simulink model "Zad_3_sch"  (R2022a)
settings: Solver=VariableStepAuto  StartTime=0.0  StopTime=10.0  RelTol=1e-3
values from neighbouring files (symbols this model uses):
  a21 = (1/(2*m))*x30^2*(FemP1/FemP2^2)*exp(-x10/FemP2)    [Zad_2.m]
  a23 = -(1/m)*x30*(FemP1/FemP2)*exp(-x10/FemP2)    [Zad_2.m]
  a31 = (1/f1)*exp(x10/f2)*(ki*u10+ci-x30)    [Zad_2.m]
  a33 = -(f2/f1)*exp(x10/f2)    [Zad_2.m]
  b31 = ki*(f2/f1)*exp(x10/f2)    [Zad_2.m]
  g = 9.81    [Zad_2.m]
  xd = d-bd    (= 0.01326)    [Zad_2.m]
libraries: slpidlib x1
settings Model: Creator=marci  LastModifiedBy=marci

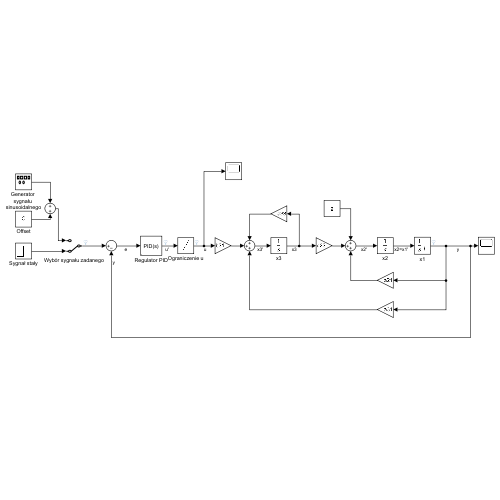
[thumbnail: Simulink's stored preview of the top-level diagram]
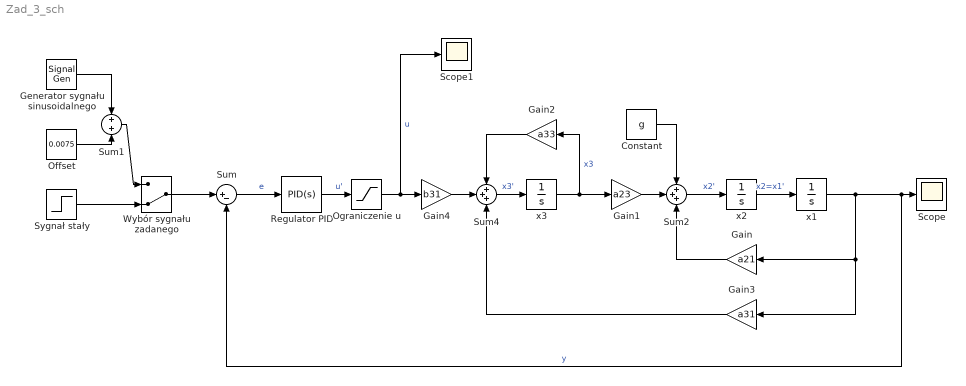
== system Zad_3_sch ==
  Constant : Constant  Value=g
  Gain : Gain  Gain=a21
  Gain1 : Gain  Gain=a23
  Gain2 : Gain  Gain=a33
  Gain3 : Gain  Gain=a31
  Gain4 : Gain  Gain=b31
  Generator sygnału sinusoidalnego : SignalGenerator  Amplitude=0.005  Frequency=4  Units=rad/sec
  Offset : Constant  Value=0.0075
  Ograniczenie u : Saturate  UpperLimit=1  LowerLimit=0
  Regulator PID : slpidlib/PID Controller  Controller=PID  Form=Parallel  TimeDomain=Continuous-time  UseExternalTs=off  SampleTime=-1  IntegratorMethod=Forward Euler  FilterMethod=Forward Euler  ControllerParametersSource=internal  P=-534.473828289694  I=-2305.65297470383  UseKiTs=off  D=-14.9649316144932  N=6018.04430338839  UseFilter=on  TunerSelectOption=Transfer Function Based (PID Tuner App)  InitialConditionSource=internal  InitialConditionForIntegrator=0  InitialConditionForFilter=0  DifferentiatorICPrevScaledInput=0  ExternalReset=none  TrackingMode=off  Kt=1  LimitOutput=off  SatLimitsSource=internal  UpperSaturationLimit=inf  LowerSaturationLimit=-inf  LinearizeAsGain=on  AntiWindupMode=none  Kb=1  POutMin=[]  POutMax=[]  IOutMin=[]  IOutMax=[]  DOutMin=[]  DOutMax=[]  NOutMin=[]  NOutMax=[]  SumOutMin=[]  SumOutMax=[]  SaturationOutMin=[]  SaturationOutMax=[]  PParamMin=[]  PParamMax=[]  IParamMin=[]  IParamMax=[]  DParamMin=[]  DParamMax=[]  NParamMin=[]  NParamMax=[]  KbParamMin=[]  KbParamMax=[]  KtParamMin=[]  KtParamMax=[]  KbOutMin=[]  KbOutMax=[]  KtOutMin=[]  KtOutMax=[]  IntegratorOutMin=[]  IntegratorOutMax=[]  FilterOutMin=[]  FilterOutMax=[]  SumI1OutMin=[]  SumI1OutMax=[]  SumI2OutMin=[]  SumI2OutMax=[]  SumI3OutMin=[]  SumI3OutMax=[]  SumI4OutMin=[]  SumI4OutMax=[]  SumDOutMin=[]  SumDOutMax=[]  DifferentiatorOutMin=[]  DifferentiatorOutMax=[]  FilterDiffOutCoefMin=[]  FilterDiffOutCoefMax=[]  ReciprocalOutMin=[]  ReciprocalOutMax=[]  SumDenOutMin=[]  SumDenOutMax=[]  SumNumOutMin=[]  SumNumOutMax=[]  DivideOutMin=[]  DivideOutMax=[]  UdiffTsProdOutMin=[]  UdiffTsProdOutMax=[]  NTsProdOutMin=[]  NTsProdOutMax=[]  UintegralTsProdOutMin=[]  UintegralTsProdOutMax=[]  UngainTsProdOutMin=[]  UngainTsProdOutMax=[]  IntegratorContinuousStateAttributes=''  IntegratorStateMustResolveToSignalObject=off  IntegratorRTWStateStorageClass=Auto  FilterContinuousStateAttributes=''  FilterStateMustResolveToSignalObject=off  FilterRTWStateStorageClass=Auto  ParallelPVariant=InternalParameters  IdealPVariant=Disabled  IVariant=InternalParameters  DVariant=InternalParameters  IntegratorVariant=Continuous  SatVariant=Disabled  AWVariant=Passthrough  PCopyVariant=Disabled  TRVariant=Disabled  FdbkBlocksVariant=Forward  IdealPFdbkVariant=Disabled  SatFdbkVariant=Disabled  DerivativeFilterVariant=ContFilter  NVariant=InternalParameters  NCopyVariant=Disabled  FilterICVariant=InternalICsFilter  IntegratorICVariant=InternalICs  ExternalResetVariant=Disabled  TRSumVariant=Passthrough  SumFdbkVariant=Disabled  SumVariant=Sum_PID  TsampFilterVariant=InternalTs  TsampNgainVariant=Passthrough  TsampIntegralVariant=Passthrough  ExternalSaturationOutDataTypeStr=Inherit: Same as second input  aMode=0
  Scope : Scope
  Scope1 : Scope
  Sum : Sum  Inputs=|+-
  Sum1 : Sum
  Sum2 : Sum  Inputs=+++
  Sum4 : Sum  Inputs=+++
  Sygnał stały : Step  Time=0  After=0.008  SampleTime=0
  Wybór sygnału zadanego : ManualSwitch  CurrentSetting=0
  x1 : Integrator  InitialCondition=xd  LimitOutput=on  UpperSaturationLimit=xd  LowerSaturationLimit=0
  x2 : Integrator
  x3 : Integrator
  wires:
  Regulator PID/1 -> Ograniczenie u/1  "u'"
  x1/1 -> Sum/2, Scope/1, Gain/1, Gain3/1  "y"
  Wybór sygnału zadanego/1 -> Sum/1
  Sum/1 -> Regulator PID/1  "e"
  Sum1/1 -> Wybór sygnału zadanego/1
  Offset/1 -> Sum1/2
  Generator sygnału sinusoidalnego/1 -> Sum1/1
  Sygnał stały/1 -> Wybór sygnału zadanego/2
  Gain3/1 -> Sum4/3
  Ograniczenie u/1 -> Scope1/1, Gain4/1  "u"
  Sum2/1 -> x2/1  "x2'"
  x3/1 -> Gain1/1, Gain2/1  "x3"
  x2/1 -> x1/1  "x2=x1'"
  Constant/1 -> Sum2/1
  Gain2/1 -> Sum4/1
  Gain/1 -> Sum2/3
  Sum4/1 -> x3/1  "x3'"
  Gain4/1 -> Sum4/2
  Gain1/1 -> Sum2/2
